simulink model "CANFDModel410_3"  (R2014a)
settings: Solver=ode45  StartTime=0.0  StopTime=200  RelTol=1e-3
undefined symbols (not defined in the file or in its folder): des, gcbh
undefined symbols (not defined in the file): BitR1, BitR2, DS, GEN_TIME
libraries: simeventslib x2, simulink x1
settings Model: Creator=PcMax  LastModifiedBy=PcMax

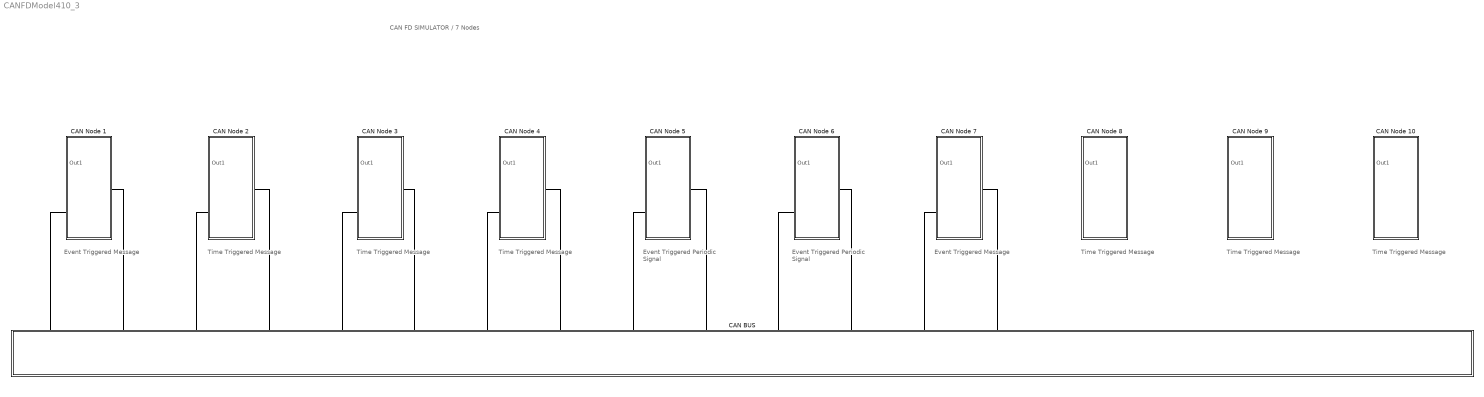
== system CANFDModel410_3 ==
  note: Event Triggered
      | Message
  note: CAN FD SIMULATOR / 7 Nodes
  note: Time Triggered
      | Message
  note: Event Triggered
      | Periodic Signal
  note: Time Triggered
      | Message
  note: Time Triggered
      | Message
  note: Event Triggered
      | Message
  note: Time Triggered
      | Message
  note: Time Triggered
      | Message
  note: Time Triggered
      | Message
  note: Event Triggered
      | Periodic Signal
  CAN BUS : Subsystem  mask{BitRate1=BitR1, BitRate2=BitR2, DSize=DS}
      mask prompts: BitRate1 "BitRate1 (Up to 1000 Kbit/s)"; BitRate2 "BitRate2 (Up to 8000 Kbit/s)"; DSize "DataSize (Up to 64 bytes)"
  CAN Node 1 : Subsystem  mask{Tint=GEN_TIME, Acc_ID=2, CAN_ID=1, bitlength=16, MAXM=800, MINM=400}
      mask prompts: Tint "Generation Time"; Acc_ID "Accepted CAN ID"; CAN_ID "Generation CAN ID"; bitlength "Bit Length"; MAXM "Message High"; MINM "Message Low"
  CAN Node 10 : Subsystem  mask{Tint=GEN_TIME, Acc_ID=2, CAN_ID=10, bitlength=16, MAXM=800, MINM=400}
      mask prompts: Tint "Generation Time"; Acc_ID "Accepted CAN ID"; CAN_ID "Generation CAN ID"; bitlength "Bit Length"; MAXM "Message High"; MINM "Message Low"
  CAN Node 2 : Subsystem  mask{Tint=GEN_TIME+5, Acc_ID=3, CAN_ID=2, bitlength=16, MAXM=800, MINM=400}
      mask prompts: Tint "Generation Time"; Acc_ID "Accepted CAN ID"; CAN_ID "Generation CAN ID"; bitlength "Bit Length"; MAXM "Message High"; MINM "Message Low"
  CAN Node 3 : Subsystem  mask{Tint=GEN_TIME+4, Acc_ID=2, CAN_ID=3, bitlength=16, MAXM=800, MINM=400}
      mask prompts: Tint "Generation Time"; Acc_ID "Accepted CAN ID"; CAN_ID "Generation CAN ID"; bitlength "Bit Length"; MAXM "Message High"; MINM "Message Low"
  CAN Node 4 : Subsystem  mask{Tint=GEN_TIME+3, Acc_ID=2, CAN_ID=4, bitlength=16, MAXM=800, MINM=400}
      mask prompts: Tint "Generation Time"; Acc_ID "Accepted CAN ID"; CAN_ID "Generation CAN ID"; bitlength "Bit Length"; MAXM "Message High"; MINM "Message Low"
  CAN Node 5 : Subsystem  mask{Tint=GEN_TIME, Acc_ID=1, CAN_ID=5, bitlength=16, MAXM=800, MINM=400}
      mask prompts: Tint "Generation Time"; Acc_ID "Accepted CAN ID"; CAN_ID "Generation CAN ID"; bitlength "Bit Length"; MAXM "Message High"; MINM "Message Low"
  CAN Node 6 : Subsystem  mask{Tint=GEN_TIME, Acc_ID=1, CAN_ID=6, bitlength=16, MAXM=800, MINM=400}
      mask prompts: Tint "Generation Time"; Acc_ID "Accepted CAN ID"; CAN_ID "Generation CAN ID"; bitlength "Bit Length"; MAXM "Message High"; MINM "Message Low"
  CAN Node 7 : Subsystem  mask{Tint=GEN_TIME, Acc_ID=2, CAN_ID=7, bitlength=16, MAXM=800, MINM=400}
      mask prompts: Tint "Generation Time"; Acc_ID "Accepted CAN ID"; CAN_ID "Generation CAN ID"; bitlength "Bit Length"; MAXM "Message High"; MINM "Message Low"
  CAN Node 8 : Subsystem  mask{Tint=GEN_TIME+2, Acc_ID=4, CAN_ID=8, bitlength=16, MAXM=800, MINM=400}
      mask prompts: Tint "Generation Time"; Acc_ID "Accepted CAN ID"; CAN_ID "Generation CAN ID"; bitlength "Bit Length"; MAXM "Message High"; MINM "Message Low"
  CAN Node 9 : Subsystem  mask{Tint=GEN_TIME+1, Acc_ID=6, CAN_ID=9, bitlength=16, MAXM=800, MINM=400}
      mask prompts: Tint "Generation Time"; Acc_ID "Accepted CAN ID"; CAN_ID "Generation CAN ID"; bitlength "Bit Length"; MAXM "Message High"; MINM "Message Low"
  connections:
  CAN Node 1/RConn1 -- CAN BUS/LConn1
  CAN Node 1/LConn1 -- CAN BUS/LConn2
  CAN Node 2/LConn1 -- CAN BUS/LConn4
  CAN BUS/LConn6 -- CAN Node 3/LConn1
  CAN Node 2/RConn1 -- CAN BUS/LConn3
  CAN Node 3/RConn1 -- CAN BUS/LConn5
  CAN Node 4/RConn1 -- CAN BUS/LConn7
  CAN Node 4/LConn1 -- CAN BUS/LConn8
  CAN Node 5/RConn1 -- CAN BUS/LConn9
  CAN Node 5/LConn1 -- CAN BUS/LConn10
  CAN Node 6/RConn1 -- CAN BUS/LConn11
  CAN Node 6/LConn1 -- CAN BUS/LConn12
  CAN Node 7/RConn1 -- CAN BUS/LConn13
  CAN Node 7/LConn1 -- CAN BUS/LConn14

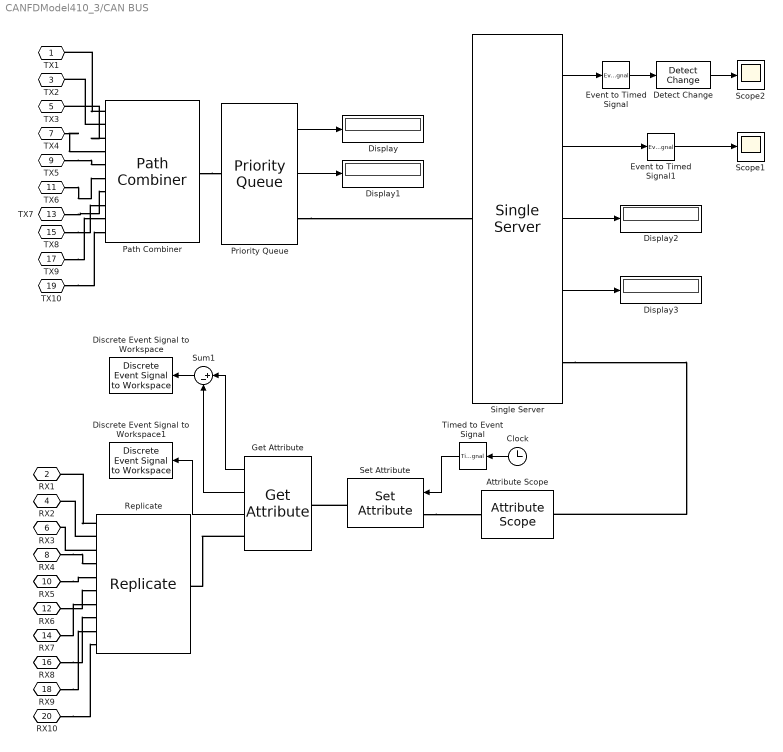
== system CANFDModel410_3/CAN BUS ==
  Attribute Scope : AttributeScope  LoadFcn=des.scope.CallbackSupport('seLoadFcn',gcbh)  StartFcn=des.scope.CallbackSupport('seStartFcn',gcbh)  StopFcn=des.scope.CallbackSupport('seStopFcn',gcbh)  PlotType=Stem  AttributeNameY=CAN_ID
      settings: CopyFcn=des.scope.CallbackSupport('seCopyFcn',gcbh)  DeleteFcn=des.scope.CallbackSupport('seDeleteFcn',gcbh)  PreSaveFcn=des.scope.CallbackSupport('sePreSaveFcn',gcbh)  NameChangeFcn=des.scope.CallbackSupport('seNameChangeFcn',gcbh)  OpenFcn=des.scope.CallbackSupport('seOpenFcn',gcbh)
  Clock : Clock
  Detect Change : simulink/Logic and Bit Operations/Detect Change  vinit=0  InputProcessing=Inherited  OutDataTypeStr=boolean
  Discrete Event Signal to Workspace : simeventslib/SimEvents Sinks/Discrete Event Signal to Workspace  VariableName=D  SaveFormat=Array  isMonitorOnly=off  isRecordIC=off
  Discrete Event Signal to Workspace1 : simeventslib/SimEvents Sinks/Discrete Event Signal to Workspace  VariableName=ID  SaveFormat=Array  isMonitorOnly=off  isRecordIC=off
  Display{,1..3} (4 alike) : Display
  Event to Timed Signal : EventToTimedSignal
  Event to Timed Signal1 : EventToTimedSignal
  Get Attribute : GetAttribute  AttributeName=Tim_arv|Tim_gen|CAN_ID  AttributeMissing=Error|Error|Error  AttributeDefaultValue=1|1|1  AttributeTreatAsVector=1|1|1  AttributeSendTiming=After entity departure|After entity departure|After entity departure  EvaluatedDefaultAttributeValue={ [];[];[]}
      settings: OutputPortMap=o1,o2,o3
  Path Combiner : PathCombiner  NumberInputPorts=10
  Priority Queue : PriorityQueue  Capacity=10  SortingAttributeName=CAN_ID  StatAverageWait=on  StatNumberTimedout=on
      settings: OutputPortMap=o2,o4
  Replicate : Replicate  NumberOutputPorts=10
  Scope1 : Scope
  Scope2 : Scope
      settings: SaveName=ScopeData2
  Set Attribute : SetAttribute  AttributeName=Tim_arv  AttributeFrom=Signal port  EvaluatedAttributeValue={ []}
  Single Server : SingleServer  ServiceTime=(32/BitRate1)+((28+10*DSize+17)/BitRate2)  StatNumberDeparted=on  StatNumberInBlock=on  StatAverageWait=on  StatUtilization=on
      settings: OutputPortMap=o0,o1,o4,o5
  Sum1 : Sum  Inputs=|+-
  Timed to Event Signal : TimedToEventSignal
  TX1 : PMIOPort  Port=1  Side=Left
  RX1 : PMIOPort  Port=2  Side=Left
  TX2 : PMIOPort  Port=3  Side=Left
  RX2 : PMIOPort  Port=4  Side=Left
  TX3 : PMIOPort  Port=5  Side=Left
  RX3 : PMIOPort  Port=6  Side=Left
  TX4 : PMIOPort  Port=7  Side=Left
  RX4 : PMIOPort  Port=8  Side=Left
  TX5 : PMIOPort  Port=9  Side=Left
  RX5 : PMIOPort  Port=10  Side=Left
  TX6 : PMIOPort  Port=11  Side=Left
  RX6 : PMIOPort  Port=12  Side=Left
  TX7 : PMIOPort  Port=13  Side=Left
  RX7 : PMIOPort  Port=14  Side=Left
  TX8 : PMIOPort  Port=15  Side=Left
  RX8 : PMIOPort  Port=16  Side=Left
  TX9 : PMIOPort  Port=17  Side=Left
  RX9 : PMIOPort  Port=18  Side=Left
  TX10 : PMIOPort  Port=19  Side=Left
  RX10 : PMIOPort  Port=20  Side=Left
  wires:
  Priority Queue/1 -> Display/1
  Single Server/4 -> Display3/1
  Single Server/1 -> Event to Timed Signal/1
  Single Server/2 -> Event to Timed Signal1/1
  Event to Timed Signal1/1 -> Scope1/1
  Priority Queue/2 -> Display1/1
  Single Server/3 -> Display2/1
  Event to Timed Signal/1 -> Detect Change/1
  Detect Change/1 -> Scope2/1
  Clock/1 -> Timed to Event Signal/1
  Timed to Event Signal/1 -> Set Attribute/1
  Get Attribute/1 -> Sum1/1
  Get Attribute/2 -> Sum1/2
  Get Attribute/3 -> Discrete Event Signal to Workspace1/1
  Sum1/1 -> Discrete Event Signal to Workspace/1
  connections:
  Path Combiner/LConn2 -- TX2/RConn1
  Replicate/RConn2 -- RX2/RConn1
  Path Combiner/LConn3 -- TX3/RConn1
  Replicate/RConn3 -- RX3/RConn1
  Path Combiner/LConn1 -- TX1/RConn1
  Replicate/RConn1 -- RX1/RConn1
  Priority Queue/RConn1 -- Single Server/LConn1
  Path Combiner/RConn1 -- Priority Queue/LConn1
  Single Server/RConn1 -- Attribute Scope/LConn1
  Set Attribute/LConn1 -- Attribute Scope/RConn1
  Set Attribute/RConn1 -- Get Attribute/LConn1
  Get Attribute/RConn1 -- Replicate/LConn1
  TX4/RConn1 -- Path Combiner/LConn4
  RX4/RConn1 -- Replicate/RConn4
  TX5/RConn1 -- Path Combiner/LConn5
  RX5/RConn1 -- Replicate/RConn5
  TX6/RConn1 -- Path Combiner/LConn6
  RX6/RConn1 -- Replicate/RConn6
  TX7/RConn1 -- Path Combiner/LConn7
  RX7/RConn1 -- Replicate/RConn7
  TX8/RConn1 -- Path Combiner/LConn8
  RX8/RConn1 -- Replicate/RConn8
  TX9/RConn1 -- Path Combiner/LConn9
  RX9/RConn1 -- Replicate/RConn9
  TX10/RConn1 -- Path Combiner/LConn10
  RX10/RConn1 -- Replicate/RConn10

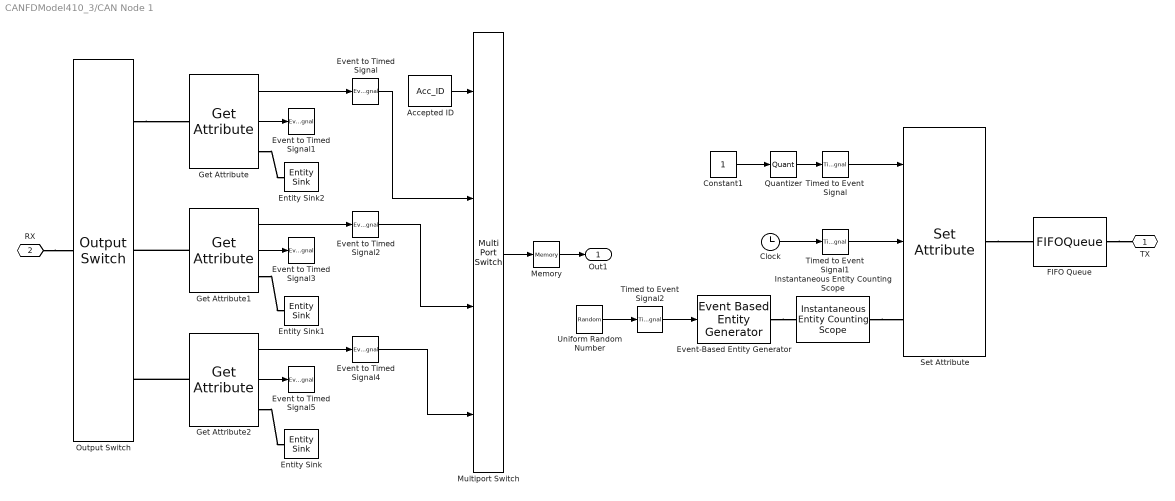
== system CANFDModel410_3/CAN Node 1 ==
  Accepted ID : Constant  Value=Acc_ID
  Clock : Clock
  Constant1 : Constant
  Entity Sink : EntitySink
  Entity Sink1 : EntitySink
  Entity Sink2 : EntitySink
  Event to Timed Signal{,1..5} (6 alike) : EventToTimedSignal
  Event-Based Entity Generator : EventBasedEntityGenerator
  FIFO Queue : FIFOQueue  Capacity=3
  Get Attribute : GetAttribute  AttributeName=Value|CAN_ID  AttributeMissing=Error|Error  AttributeDefaultValue=1|1  AttributeTreatAsVector=1|1  AttributeSendTiming=After entity departure|After entity departure  EvaluatedDefaultAttributeValue={ [];[]}
      settings: OutputPortMap=o1,o2
  Get Attribute1 : GetAttribute  AttributeName=Value|CAN_ID  AttributeMissing=Error|Error  AttributeDefaultValue=1|1  AttributeTreatAsVector=1|1  AttributeSendTiming=After entity departure|After entity departure  EvaluatedDefaultAttributeValue={ [];[]}
      settings: OutputPortMap=o1,o2
  Get Attribute2 : GetAttribute  AttributeName=Value|CAN_ID  AttributeMissing=Error|Error  AttributeDefaultValue=1|1  AttributeTreatAsVector=1|1  AttributeSendTiming=After entity departure|After entity departure  EvaluatedDefaultAttributeValue={ [];[]}
      settings: OutputPortMap=o1,o2
  Instantaneous Entity Counting Scope : InstantaneousEntityCountingScope  LoadFcn=des.scope.CallbackSupport('seLoadFcn',gcbh)  StartFcn=des.scope.CallbackSupport('seStartFcn',gcbh)  StopFcn=des.scope.CallbackSupport('seStopFcn',gcbh)
      settings: CopyFcn=des.scope.CallbackSupport('seCopyFcn',gcbh)  DeleteFcn=des.scope.CallbackSupport('seDeleteFcn',gcbh)  PreSaveFcn=des.scope.CallbackSupport('sePreSaveFcn',gcbh)  NameChangeFcn=des.scope.CallbackSupport('seNameChangeFcn',gcbh)  OpenFcn=des.scope.CallbackSupport('seOpenFcn',gcbh)
  Memory : Memory
  Multiport Switch : MultiPortSwitch
  Output Switch : OutputSwitch
  Quantizer : Quantizer  QuantizationInterval=(MAXM-MINM)/2^bitlength%%800/2^16%%
  Set Attribute : SetAttribute  AttributeName=Value|Tim_gen|CAN_ID  AttributeFrom=Signal port|Signal port|Dialog  AttributeValue=1|1|CAN_ID  AttributeTreatAsVector=1|1|1  EvaluatedAttributeValue={ [];[];CAN_ID}
      settings: InputPortMap=u0,u1
  Timed to Event Signal : TimedToEventSignal
  Timed to Event Signal1 : TimedToEventSignal
  Timed to Event Signal2 : TimedToEventSignal
  Uniform Random Number : UniformRandomNumber  SampleTime=Tint + 4
  TX : PMIOPort  Port=1  Side=Right
  RX : PMIOPort  Port=2  Side=Left
  Out1 : Outport
  wires:
  Quantizer/1 -> Timed to Event Signal/1
  Timed to Event Signal/1 -> Set Attribute/1
  Clock/1 -> Timed to Event Signal1/1
  Timed to Event Signal1/1 -> Set Attribute/2
  Constant1/1 -> Quantizer/1
  Get Attribute/2 -> Event to Timed Signal1/1
  Get Attribute/1 -> Event to Timed Signal/1
  Get Attribute1/1 -> Event to Timed Signal2/1
  Get Attribute1/2 -> Event to Timed Signal3/1
  Get Attribute2/1 -> Event to Timed Signal4/1
  Get Attribute2/2 -> Event to Timed Signal5/1
  Event to Timed Signal/1 -> Multiport Switch/2
  Event to Timed Signal2/1 -> Multiport Switch/3
  Event to Timed Signal4/1 -> Multiport Switch/4
  Accepted ID/1 -> Multiport Switch/1
  Multiport Switch/1 -> Memory/1
  Uniform Random Number/1 -> Timed to Event Signal2/1
  Timed to Event Signal2/1 -> Event-Based Entity Generator/1
  Memory/1 -> Out1/1
  connections:
  Set Attribute/RConn1 -- FIFO Queue/LConn1
  Event-Based Entity Generator/RConn1 -- Instantaneous Entity Counting Scope/LConn1
  FIFO Queue/RConn1 -- TX/RConn1
  RX/RConn1 -- Output Switch/LConn1
  Output Switch/RConn1 -- Get Attribute/LConn1
  Get Attribute1/LConn1 -- Output Switch/RConn2
  Get Attribute2/LConn1 -- Output Switch/RConn3
  Get Attribute2/RConn1 -- Entity Sink/LConn1
  Get Attribute/RConn1 -- Entity Sink2/LConn1
  Get Attribute1/RConn1 -- Entity Sink1/LConn1
  Instantaneous Entity Counting Scope/RConn1 -- Set Attribute/LConn1

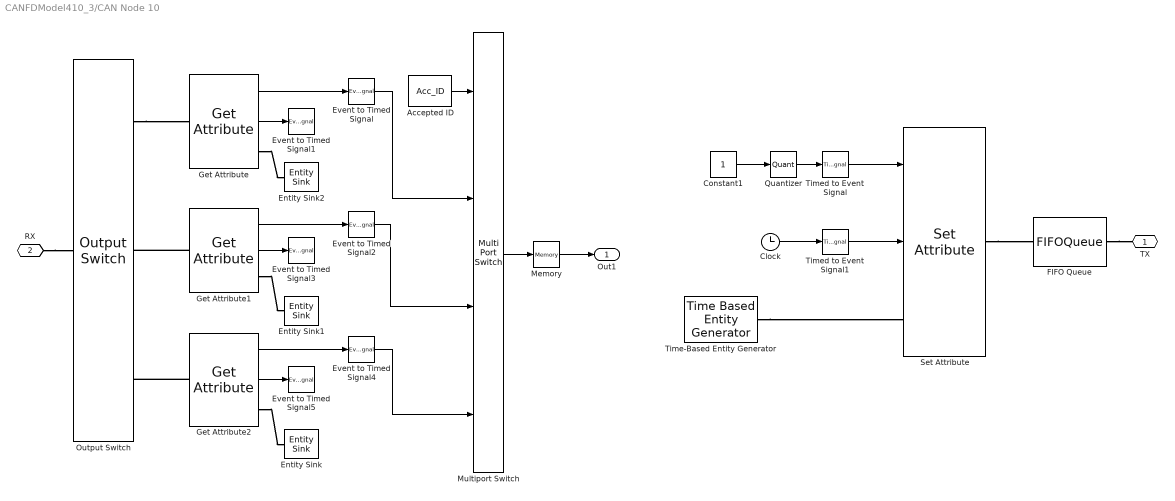
== system CANFDModel410_3/CAN Node 10 ==
  Accepted ID : Constant  Value=Acc_ID
  Clock : Clock
  Constant1 : Constant
  Entity Sink : EntitySink
  Entity Sink1 : EntitySink
  Entity Sink2 : EntitySink
  Event to Timed Signal{,1..5} (6 alike) : EventToTimedSignal
  FIFO Queue : FIFOQueue  Capacity=3
  Get Attribute : GetAttribute  AttributeName=Value|CAN_ID  AttributeMissing=Error|Error  AttributeDefaultValue=1|1  AttributeTreatAsVector=1|1  AttributeSendTiming=After entity departure|After entity departure  EvaluatedDefaultAttributeValue={ [];[]}
      settings: OutputPortMap=o1,o2
  Get Attribute1 : GetAttribute  AttributeName=Value|CAN_ID  AttributeMissing=Error|Error  AttributeDefaultValue=1|1  AttributeTreatAsVector=1|1  AttributeSendTiming=After entity departure|After entity departure  EvaluatedDefaultAttributeValue={ [];[]}
      settings: OutputPortMap=o1,o2
  Get Attribute2 : GetAttribute  AttributeName=Value|CAN_ID  AttributeMissing=Error|Error  AttributeDefaultValue=1|1  AttributeTreatAsVector=1|1  AttributeSendTiming=After entity departure|After entity departure  EvaluatedDefaultAttributeValue={ [];[]}
      settings: OutputPortMap=o1,o2
  Memory : Memory
  Multiport Switch : MultiPortSwitch
  Output Switch : OutputSwitch
  Quantizer : Quantizer  QuantizationInterval=(MAXM-MINM)/2^bitlength%%800/2^16%%
  Set Attribute : SetAttribute  AttributeName=Value|Tim_gen|CAN_ID  AttributeFrom=Signal port|Signal port|Dialog  AttributeValue=1|1|CAN_ID  AttributeTreatAsVector=1|1|1  EvaluatedAttributeValue={ [];[];CAN_ID}
      settings: InputPortMap=u0,u1
  Time-Based Entity Generator : TimeBasedEntityGenerator  Distribution=Uniform  Period=Tint  Minimum=Tint  Maximum=Tint+0.1
  Timed to Event Signal : TimedToEventSignal
  Timed to Event Signal1 : TimedToEventSignal
  TX : PMIOPort  Port=1  Side=Right
  RX : PMIOPort  Port=2  Side=Left
  Out1 : Outport
  wires:
  Quantizer/1 -> Timed to Event Signal/1
  Timed to Event Signal/1 -> Set Attribute/1
  Clock/1 -> Timed to Event Signal1/1
  Timed to Event Signal1/1 -> Set Attribute/2
  Constant1/1 -> Quantizer/1
  Get Attribute/2 -> Event to Timed Signal1/1
  Get Attribute/1 -> Event to Timed Signal/1
  Get Attribute1/1 -> Event to Timed Signal2/1
  Get Attribute1/2 -> Event to Timed Signal3/1
  Get Attribute2/1 -> Event to Timed Signal4/1
  Get Attribute2/2 -> Event to Timed Signal5/1
  Event to Timed Signal/1 -> Multiport Switch/2
  Event to Timed Signal2/1 -> Multiport Switch/3
  Event to Timed Signal4/1 -> Multiport Switch/4
  Accepted ID/1 -> Multiport Switch/1
  Multiport Switch/1 -> Memory/1
  Memory/1 -> Out1/1
  connections:
  Set Attribute/RConn1 -- FIFO Queue/LConn1
  Time-Based Entity Generator/RConn1 -- Set Attribute/LConn1
  FIFO Queue/RConn1 -- TX/RConn1
  RX/RConn1 -- Output Switch/LConn1
  Output Switch/RConn1 -- Get Attribute/LConn1
  Get Attribute1/LConn1 -- Output Switch/RConn2
  Get Attribute2/LConn1 -- Output Switch/RConn3
  Get Attribute2/RConn1 -- Entity Sink/LConn1
  Get Attribute/RConn1 -- Entity Sink2/LConn1
  Get Attribute1/RConn1 -- Entity Sink1/LConn1

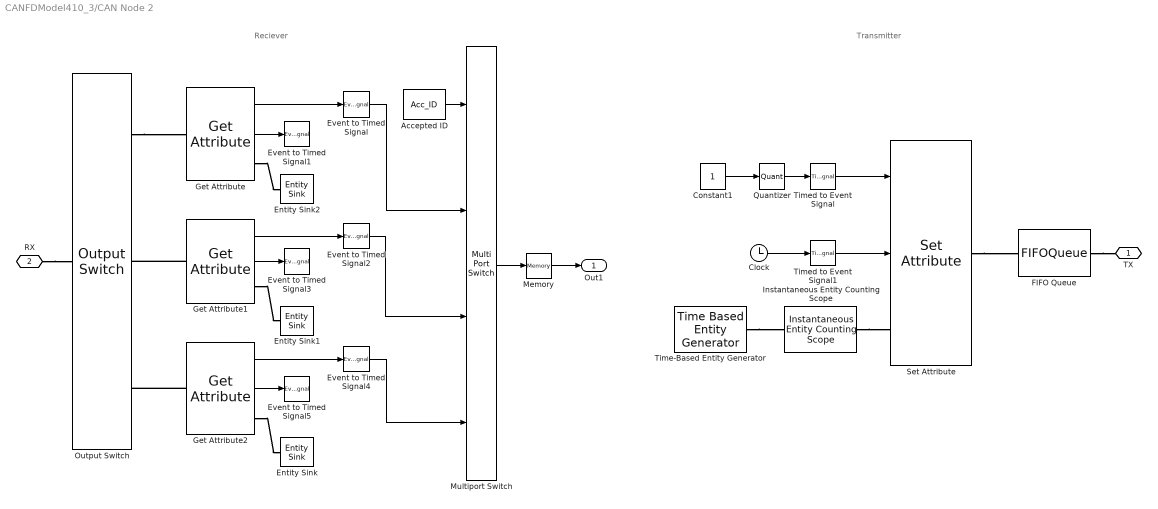
== system CANFDModel410_3/CAN Node 2 ==
  note: Reciever
  note: Transmitter
  Accepted ID : Constant  Value=Acc_ID
  Clock : Clock
  Constant1 : Constant
  Entity Sink : EntitySink
  Entity Sink1 : EntitySink
  Entity Sink2 : EntitySink
  Event to Timed Signal{,1..5} (6 alike) : EventToTimedSignal
  FIFO Queue : FIFOQueue  Capacity=3
  Get Attribute : GetAttribute  AttributeName=Value|CAN_ID  AttributeMissing=Error|Error  AttributeDefaultValue=1|1  AttributeTreatAsVector=1|1  AttributeSendTiming=After entity departure|After entity departure  EvaluatedDefaultAttributeValue={ [];[]}
      settings: OutputPortMap=o1,o2
  Get Attribute1 : GetAttribute  AttributeName=Value|CAN_ID  AttributeMissing=Error|Error  AttributeDefaultValue=1|1  AttributeTreatAsVector=1|1  AttributeSendTiming=After entity departure|After entity departure  EvaluatedDefaultAttributeValue={ [];[]}
      settings: OutputPortMap=o1,o2
  Get Attribute2 : GetAttribute  AttributeName=Value|CAN_ID  AttributeMissing=Error|Error  AttributeDefaultValue=1|1  AttributeTreatAsVector=1|1  AttributeSendTiming=After entity departure|After entity departure  EvaluatedDefaultAttributeValue={ [];[]}
      settings: OutputPortMap=o1,o2
  Instantaneous Entity Counting Scope : InstantaneousEntityCountingScope  LoadFcn=des.scope.CallbackSupport('seLoadFcn',gcbh)  StartFcn=des.scope.CallbackSupport('seStartFcn',gcbh)  StopFcn=des.scope.CallbackSupport('seStopFcn',gcbh)
      settings: CopyFcn=des.scope.CallbackSupport('seCopyFcn',gcbh)  DeleteFcn=des.scope.CallbackSupport('seDeleteFcn',gcbh)  PreSaveFcn=des.scope.CallbackSupport('sePreSaveFcn',gcbh)  NameChangeFcn=des.scope.CallbackSupport('seNameChangeFcn',gcbh)  OpenFcn=des.scope.CallbackSupport('seOpenFcn',gcbh)
  Memory : Memory
  Multiport Switch : MultiPortSwitch
  Output Switch : OutputSwitch
  Quantizer : Quantizer  QuantizationInterval=(MAXM-MINM)/2^bitlength%%800/2^16%%
  Set Attribute : SetAttribute  AttributeName=Value|Tim_gen|CAN_ID  AttributeFrom=Signal port|Signal port|Dialog  AttributeValue=1|1|CAN_ID  AttributeTreatAsVector=1|1|1  EvaluatedAttributeValue={ [];[];CAN_ID}
      settings: InputPortMap=u0,u1
  Time-Based Entity Generator : TimeBasedEntityGenerator  Distribution=Uniform  Period=Tint  Minimum=Tint  Maximum=Tint+0.1
  Timed to Event Signal : TimedToEventSignal
  Timed to Event Signal1 : TimedToEventSignal
  TX : PMIOPort  Port=1  Side=Right
  RX : PMIOPort  Port=2  Side=Left
  Out1 : Outport
  wires:
  Memory/1 -> Out1/1
  Multiport Switch/1 -> Memory/1
  Accepted ID/1 -> Multiport Switch/1
  Event to Timed Signal4/1 -> Multiport Switch/4
  Event to Timed Signal2/1 -> Multiport Switch/3
  Event to Timed Signal/1 -> Multiport Switch/2
  Get Attribute2/2 -> Event to Timed Signal5/1
  Get Attribute2/1 -> Event to Timed Signal4/1
  Get Attribute1/2 -> Event to Timed Signal3/1
  Get Attribute1/1 -> Event to Timed Signal2/1
  Get Attribute/1 -> Event to Timed Signal/1
  Get Attribute/2 -> Event to Timed Signal1/1
  Constant1/1 -> Quantizer/1
  Timed to Event Signal1/1 -> Set Attribute/2
  Clock/1 -> Timed to Event Signal1/1
  Timed to Event Signal/1 -> Set Attribute/1
  Quantizer/1 -> Timed to Event Signal/1
  connections:
  Get Attribute1/RConn1 -- Entity Sink1/LConn1
  Get Attribute/RConn1 -- Entity Sink2/LConn1
  Get Attribute2/RConn1 -- Entity Sink/LConn1
  Get Attribute2/LConn1 -- Output Switch/RConn3
  Get Attribute1/LConn1 -- Output Switch/RConn2
  Output Switch/RConn1 -- Get Attribute/LConn1
  RX/RConn1 -- Output Switch/LConn1
  FIFO Queue/RConn1 -- TX/RConn1
  Time-Based Entity Generator/RConn1 -- Instantaneous Entity Counting Scope/LConn1
  Set Attribute/RConn1 -- FIFO Queue/LConn1
  Instantaneous Entity Counting Scope/RConn1 -- Set Attribute/LConn1

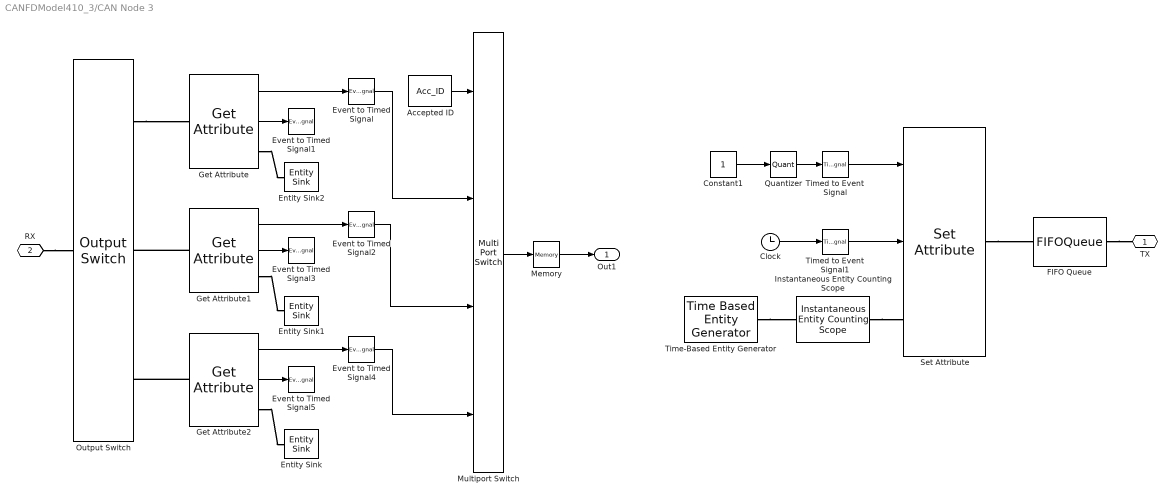
== system CANFDModel410_3/CAN Node 3 ==
  Accepted ID : Constant  Value=Acc_ID
  Clock : Clock
  Constant1 : Constant
  Entity Sink : EntitySink
  Entity Sink1 : EntitySink
  Entity Sink2 : EntitySink
  Event to Timed Signal{,1..5} (6 alike) : EventToTimedSignal
  FIFO Queue : FIFOQueue  Capacity=3
  Get Attribute : GetAttribute  AttributeName=Value|CAN_ID  AttributeMissing=Error|Error  AttributeDefaultValue=1|1  AttributeTreatAsVector=1|1  AttributeSendTiming=After entity departure|After entity departure  EvaluatedDefaultAttributeValue={ [];[]}
      settings: OutputPortMap=o1,o2
  Get Attribute1 : GetAttribute  AttributeName=Value|CAN_ID  AttributeMissing=Error|Error  AttributeDefaultValue=1|1  AttributeTreatAsVector=1|1  AttributeSendTiming=After entity departure|After entity departure  EvaluatedDefaultAttributeValue={ [];[]}
      settings: OutputPortMap=o1,o2
  Get Attribute2 : GetAttribute  AttributeName=Value|CAN_ID  AttributeMissing=Error|Error  AttributeDefaultValue=1|1  AttributeTreatAsVector=1|1  AttributeSendTiming=After entity departure|After entity departure  EvaluatedDefaultAttributeValue={ [];[]}
      settings: OutputPortMap=o1,o2
  Instantaneous Entity Counting Scope : InstantaneousEntityCountingScope  LoadFcn=des.scope.CallbackSupport('seLoadFcn',gcbh)  StartFcn=des.scope.CallbackSupport('seStartFcn',gcbh)  StopFcn=des.scope.CallbackSupport('seStopFcn',gcbh)
      settings: CopyFcn=des.scope.CallbackSupport('seCopyFcn',gcbh)  DeleteFcn=des.scope.CallbackSupport('seDeleteFcn',gcbh)  PreSaveFcn=des.scope.CallbackSupport('sePreSaveFcn',gcbh)  NameChangeFcn=des.scope.CallbackSupport('seNameChangeFcn',gcbh)  OpenFcn=des.scope.CallbackSupport('seOpenFcn',gcbh)
  Memory : Memory
  Multiport Switch : MultiPortSwitch
  Output Switch : OutputSwitch
  Quantizer : Quantizer  QuantizationInterval=(MAXM-MINM)/2^bitlength%%800/2^16%%
  Set Attribute : SetAttribute  AttributeName=Value|Tim_gen|CAN_ID  AttributeFrom=Signal port|Signal port|Dialog  AttributeValue=1|1|CAN_ID  AttributeTreatAsVector=1|1|1  EvaluatedAttributeValue={ [];[];CAN_ID}
      settings: InputPortMap=u0,u1
  Time-Based Entity Generator : TimeBasedEntityGenerator  Distribution=Uniform  Period=Tint  Minimum=Tint  Maximum=Tint+0.1
  Timed to Event Signal : TimedToEventSignal
  Timed to Event Signal1 : TimedToEventSignal
  TX : PMIOPort  Port=1  Side=Right
  RX : PMIOPort  Port=2  Side=Left
  Out1 : Outport
  wires:
  Quantizer/1 -> Timed to Event Signal/1
  Timed to Event Signal/1 -> Set Attribute/1
  Clock/1 -> Timed to Event Signal1/1
  Timed to Event Signal1/1 -> Set Attribute/2
  Constant1/1 -> Quantizer/1
  Get Attribute/2 -> Event to Timed Signal1/1
  Get Attribute/1 -> Event to Timed Signal/1
  Get Attribute1/1 -> Event to Timed Signal2/1
  Get Attribute1/2 -> Event to Timed Signal3/1
  Get Attribute2/1 -> Event to Timed Signal4/1
  Get Attribute2/2 -> Event to Timed Signal5/1
  Event to Timed Signal/1 -> Multiport Switch/2
  Event to Timed Signal2/1 -> Multiport Switch/3
  Event to Timed Signal4/1 -> Multiport Switch/4
  Accepted ID/1 -> Multiport Switch/1
  Multiport Switch/1 -> Memory/1
  Memory/1 -> Out1/1
  connections:
  Set Attribute/RConn1 -- FIFO Queue/LConn1
  Time-Based Entity Generator/RConn1 -- Instantaneous Entity Counting Scope/LConn1
  FIFO Queue/RConn1 -- TX/RConn1
  RX/RConn1 -- Output Switch/LConn1
  Output Switch/RConn1 -- Get Attribute/LConn1
  Get Attribute1/LConn1 -- Output Switch/RConn2
  Get Attribute2/LConn1 -- Output Switch/RConn3
  Get Attribute2/RConn1 -- Entity Sink/LConn1
  Get Attribute/RConn1 -- Entity Sink2/LConn1
  Get Attribute1/RConn1 -- Entity Sink1/LConn1
  Instantaneous Entity Counting Scope/RConn1 -- Set Attribute/LConn1

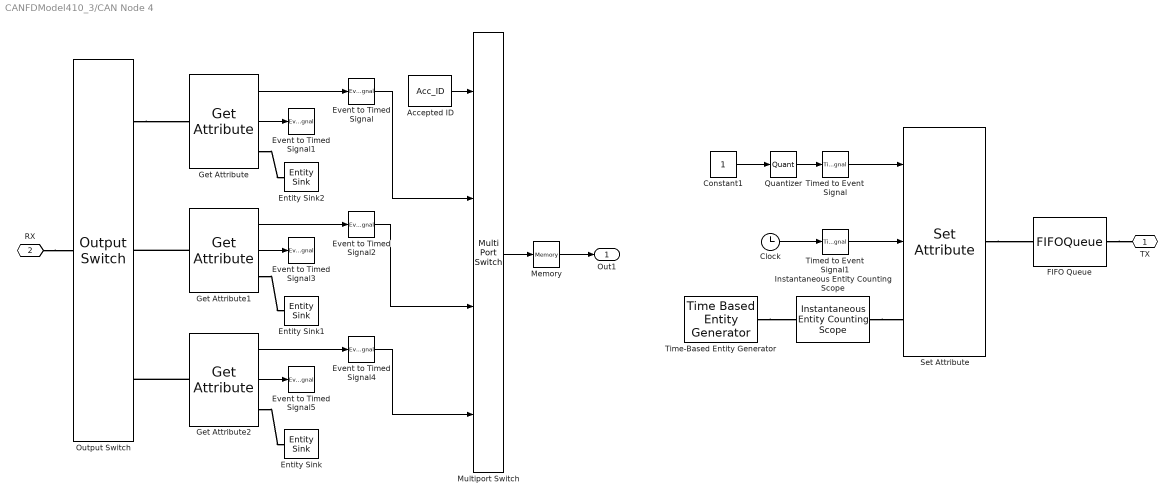
== system CANFDModel410_3/CAN Node 4 ==
  Accepted ID : Constant  Value=Acc_ID
  Clock : Clock
  Constant1 : Constant
  Entity Sink : EntitySink
  Entity Sink1 : EntitySink
  Entity Sink2 : EntitySink
  Event to Timed Signal{,1..5} (6 alike) : EventToTimedSignal
  FIFO Queue : FIFOQueue  Capacity=3
  Get Attribute : GetAttribute  AttributeName=Value|CAN_ID  AttributeMissing=Error|Error  AttributeDefaultValue=1|1  AttributeTreatAsVector=1|1  AttributeSendTiming=After entity departure|After entity departure  EvaluatedDefaultAttributeValue={ [];[]}
      settings: OutputPortMap=o1,o2
  Get Attribute1 : GetAttribute  AttributeName=Value|CAN_ID  AttributeMissing=Error|Error  AttributeDefaultValue=1|1  AttributeTreatAsVector=1|1  AttributeSendTiming=After entity departure|After entity departure  EvaluatedDefaultAttributeValue={ [];[]}
      settings: OutputPortMap=o1,o2
  Get Attribute2 : GetAttribute  AttributeName=Value|CAN_ID  AttributeMissing=Error|Error  AttributeDefaultValue=1|1  AttributeTreatAsVector=1|1  AttributeSendTiming=After entity departure|After entity departure  EvaluatedDefaultAttributeValue={ [];[]}
      settings: OutputPortMap=o1,o2
  Instantaneous Entity Counting Scope : InstantaneousEntityCountingScope  LoadFcn=des.scope.CallbackSupport('seLoadFcn',gcbh)  StartFcn=des.scope.CallbackSupport('seStartFcn',gcbh)  StopFcn=des.scope.CallbackSupport('seStopFcn',gcbh)
      settings: CopyFcn=des.scope.CallbackSupport('seCopyFcn',gcbh)  DeleteFcn=des.scope.CallbackSupport('seDeleteFcn',gcbh)  PreSaveFcn=des.scope.CallbackSupport('sePreSaveFcn',gcbh)  NameChangeFcn=des.scope.CallbackSupport('seNameChangeFcn',gcbh)  OpenFcn=des.scope.CallbackSupport('seOpenFcn',gcbh)
  Memory : Memory
  Multiport Switch : MultiPortSwitch
  Output Switch : OutputSwitch
  Quantizer : Quantizer  QuantizationInterval=(MAXM-MINM)/2^bitlength%%800/2^16%%
  Set Attribute : SetAttribute  AttributeName=Value|Tim_gen|CAN_ID  AttributeFrom=Signal port|Signal port|Dialog  AttributeValue=1|1|CAN_ID  AttributeTreatAsVector=1|1|1  EvaluatedAttributeValue={ [];[];CAN_ID}
      settings: InputPortMap=u0,u1
  Time-Based Entity Generator : TimeBasedEntityGenerator  Distribution=Uniform  Period=Tint  Minimum=Tint  Maximum=Tint+0.1
  Timed to Event Signal : TimedToEventSignal
  Timed to Event Signal1 : TimedToEventSignal
  TX : PMIOPort  Port=1  Side=Right
  RX : PMIOPort  Port=2  Side=Left
  Out1 : Outport
  wires:
  Memory/1 -> Out1/1
  Multiport Switch/1 -> Memory/1
  Accepted ID/1 -> Multiport Switch/1
  Event to Timed Signal4/1 -> Multiport Switch/4
  Event to Timed Signal2/1 -> Multiport Switch/3
  Event to Timed Signal/1 -> Multiport Switch/2
  Get Attribute2/2 -> Event to Timed Signal5/1
  Get Attribute2/1 -> Event to Timed Signal4/1
  Get Attribute1/2 -> Event to Timed Signal3/1
  Get Attribute1/1 -> Event to Timed Signal2/1
  Get Attribute/1 -> Event to Timed Signal/1
  Get Attribute/2 -> Event to Timed Signal1/1
  Constant1/1 -> Quantizer/1
  Timed to Event Signal1/1 -> Set Attribute/2
  Clock/1 -> Timed to Event Signal1/1
  Timed to Event Signal/1 -> Set Attribute/1
  Quantizer/1 -> Timed to Event Signal/1
  connections:
  Get Attribute1/RConn1 -- Entity Sink1/LConn1
  Get Attribute/RConn1 -- Entity Sink2/LConn1
  Get Attribute2/RConn1 -- Entity Sink/LConn1
  Get Attribute2/LConn1 -- Output Switch/RConn3
  Get Attribute1/LConn1 -- Output Switch/RConn2
  Output Switch/RConn1 -- Get Attribute/LConn1
  RX/RConn1 -- Output Switch/LConn1
  FIFO Queue/RConn1 -- TX/RConn1
  Instantaneous Entity Counting Scope/RConn1 -- Set Attribute/LConn1
  Set Attribute/RConn1 -- FIFO Queue/LConn1
  Time-Based Entity Generator/RConn1 -- Instantaneous Entity Counting Scope/LConn1

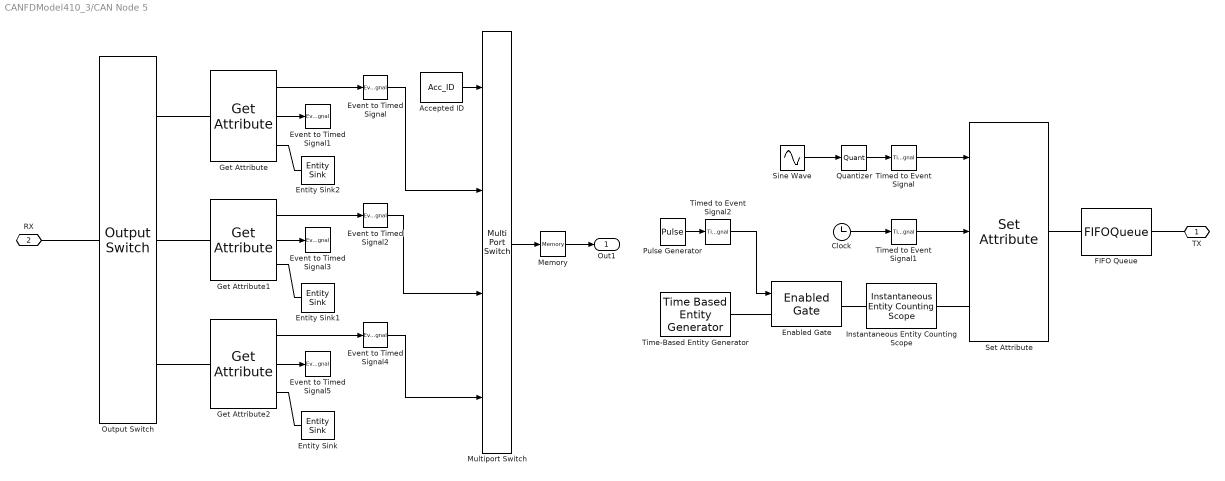
== system CANFDModel410_3/CAN Node 5 ==
  Accepted ID : Constant  Value=Acc_ID
  Clock : Clock
  Enabled Gate : EnabledGate
  Entity Sink : EntitySink
  Entity Sink1 : EntitySink
  Entity Sink2 : EntitySink
  Event to Timed Signal{,1..5} (6 alike) : EventToTimedSignal
  FIFO Queue : FIFOQueue  Capacity=3
  Get Attribute : GetAttribute  AttributeName=Value|Tim_gen  AttributeMissing=Error|Error  AttributeDefaultValue=1|1  AttributeTreatAsVector=1|1  AttributeSendTiming=After entity departure|After entity departure  EvaluatedDefaultAttributeValue={ [];[]}
      settings: OutputPortMap=o1,o2
  Get Attribute1 : GetAttribute  AttributeName=Value|Tim_gen  AttributeMissing=Error|Error  AttributeDefaultValue=1|1  AttributeTreatAsVector=1|1  AttributeSendTiming=After entity departure|After entity departure  EvaluatedDefaultAttributeValue={ [];[]}
      settings: OutputPortMap=o1,o2
  Get Attribute2 : GetAttribute  AttributeName=Value|Tim_gen  AttributeMissing=Error|Error  AttributeDefaultValue=1|1  AttributeTreatAsVector=1|1  AttributeSendTiming=After entity departure|After entity departure  EvaluatedDefaultAttributeValue={ [];[]}
      settings: OutputPortMap=o1,o2
  Instantaneous Entity Counting Scope : InstantaneousEntityCountingScope  LoadFcn=des.scope.CallbackSupport('seLoadFcn',gcbh)  StartFcn=des.scope.CallbackSupport('seStartFcn',gcbh)  StopFcn=des.scope.CallbackSupport('seStopFcn',gcbh)
      settings: CopyFcn=des.scope.CallbackSupport('seCopyFcn',gcbh)  DeleteFcn=des.scope.CallbackSupport('seDeleteFcn',gcbh)  PreSaveFcn=des.scope.CallbackSupport('sePreSaveFcn',gcbh)  NameChangeFcn=des.scope.CallbackSupport('seNameChangeFcn',gcbh)  OpenFcn=des.scope.CallbackSupport('seOpenFcn',gcbh)
  Memory : Memory
  Multiport Switch : MultiPortSwitch
  Output Switch : OutputSwitch
  Pulse Generator : DiscretePulseGenerator  Period=50  PulseWidth=30  PhaseDelay=3  VectorParams1D=off
  Quantizer : Quantizer  QuantizationInterval=(MAXM-MINM)/2^bitlength%%800/2^16%%
  Set Attribute : SetAttribute  AttributeName=Value|Tim_gen|CAN_ID  AttributeFrom=Signal port|Signal port|Dialog  AttributeValue=1|1|CAN_ID  AttributeTreatAsVector=1|1|1  EvaluatedAttributeValue={ [];[];CAN_ID}
      settings: InputPortMap=u0,u1
  Sine Wave : Sin  SampleTime=0
  Time-Based Entity Generator : TimeBasedEntityGenerator  Distribution=Uniform  Period=Tint  Minimum=Tint  Maximum=Tint+0.1  ResponseWhenUnblocked=Delayed restart
  Timed to Event Signal : TimedToEventSignal
  Timed to Event Signal1 : TimedToEventSignal
  Timed to Event Signal2 : TimedToEventSignal
  TX : PMIOPort  Port=1  Side=Right
  RX : PMIOPort  Port=2  Side=Left
  Out1 : Outport
  wires:
  Pulse Generator/1 -> Timed to Event Signal2/1
  Timed to Event Signal2/1 -> Enabled Gate/1
  Quantizer/1 -> Timed to Event Signal/1
  Timed to Event Signal/1 -> Set Attribute/1
  Clock/1 -> Timed to Event Signal1/1
  Timed to Event Signal1/1 -> Set Attribute/2
  Sine Wave/1 -> Quantizer/1
  Get Attribute/2 -> Event to Timed Signal1/1
  Get Attribute/1 -> Event to Timed Signal/1
  Get Attribute1/1 -> Event to Timed Signal2/1
  Get Attribute1/2 -> Event to Timed Signal3/1
  Get Attribute2/1 -> Event to Timed Signal4/1
  Get Attribute2/2 -> Event to Timed Signal5/1
  Event to Timed Signal/1 -> Multiport Switch/2
  Event to Timed Signal2/1 -> Multiport Switch/3
  Event to Timed Signal4/1 -> Multiport Switch/4
  Accepted ID/1 -> Multiport Switch/1
  Multiport Switch/1 -> Memory/1
  Memory/1 -> Out1/1
  connections:
  Time-Based Entity Generator/RConn1 -- Enabled Gate/LConn1
  RX/RConn1 -- Output Switch/LConn1
  Set Attribute/RConn1 -- FIFO Queue/LConn1
  Instantaneous Entity Counting Scope/LConn1 -- Enabled Gate/RConn1
  FIFO Queue/RConn1 -- TX/RConn1
  Output Switch/RConn1 -- Get Attribute/LConn1
  Get Attribute1/LConn1 -- Output Switch/RConn2
  Get Attribute2/LConn1 -- Output Switch/RConn3
  Get Attribute2/RConn1 -- Entity Sink/LConn1
  Get Attribute/RConn1 -- Entity Sink2/LConn1
  Get Attribute1/RConn1 -- Entity Sink1/LConn1
  Instantaneous Entity Counting Scope/RConn1 -- Set Attribute/LConn1

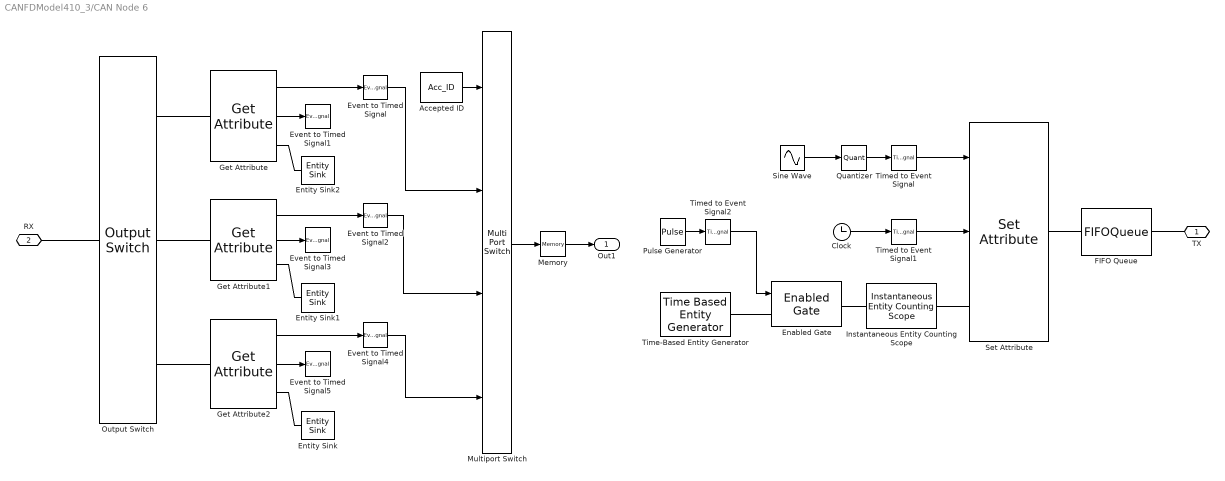
== system CANFDModel410_3/CAN Node 6 ==
  Accepted ID : Constant  Value=Acc_ID
  Clock : Clock
  Enabled Gate : EnabledGate
  Entity Sink : EntitySink
  Entity Sink1 : EntitySink
  Entity Sink2 : EntitySink
  Event to Timed Signal{,1..5} (6 alike) : EventToTimedSignal
  FIFO Queue : FIFOQueue  Capacity=3
  Get Attribute : GetAttribute  AttributeName=Value|Tim_gen  AttributeMissing=Error|Error  AttributeDefaultValue=1|1  AttributeTreatAsVector=1|1  AttributeSendTiming=After entity departure|After entity departure  EvaluatedDefaultAttributeValue={ [];[]}
      settings: OutputPortMap=o1,o2
  Get Attribute1 : GetAttribute  AttributeName=Value|Tim_gen  AttributeMissing=Error|Error  AttributeDefaultValue=1|1  AttributeTreatAsVector=1|1  AttributeSendTiming=After entity departure|After entity departure  EvaluatedDefaultAttributeValue={ [];[]}
      settings: OutputPortMap=o1,o2
  Get Attribute2 : GetAttribute  AttributeName=Value|Tim_gen  AttributeMissing=Error|Error  AttributeDefaultValue=1|1  AttributeTreatAsVector=1|1  AttributeSendTiming=After entity departure|After entity departure  EvaluatedDefaultAttributeValue={ [];[]}
      settings: OutputPortMap=o1,o2
  Instantaneous Entity Counting Scope : InstantaneousEntityCountingScope  LoadFcn=des.scope.CallbackSupport('seLoadFcn',gcbh)  StartFcn=des.scope.CallbackSupport('seStartFcn',gcbh)  StopFcn=des.scope.CallbackSupport('seStopFcn',gcbh)
      settings: CopyFcn=des.scope.CallbackSupport('seCopyFcn',gcbh)  DeleteFcn=des.scope.CallbackSupport('seDeleteFcn',gcbh)  PreSaveFcn=des.scope.CallbackSupport('sePreSaveFcn',gcbh)  NameChangeFcn=des.scope.CallbackSupport('seNameChangeFcn',gcbh)  OpenFcn=des.scope.CallbackSupport('seOpenFcn',gcbh)
  Memory : Memory
  Multiport Switch : MultiPortSwitch
  Output Switch : OutputSwitch
  Pulse Generator : DiscretePulseGenerator  Period=50  PulseWidth=30  PhaseDelay=3  VectorParams1D=off
  Quantizer : Quantizer  QuantizationInterval=(MAXM-MINM)/2^bitlength%%800/2^16%%
  Set Attribute : SetAttribute  AttributeName=Value|Tim_gen|CAN_ID  AttributeFrom=Signal port|Signal port|Dialog  AttributeValue=1|1|CAN_ID  AttributeTreatAsVector=1|1|1  EvaluatedAttributeValue={ [];[];CAN_ID}
      settings: InputPortMap=u0,u1
  Sine Wave : Sin  SampleTime=0
  Time-Based Entity Generator : TimeBasedEntityGenerator  Distribution=Uniform  Period=Tint  Minimum=Tint  Maximum=Tint+0.1  ResponseWhenUnblocked=Delayed restart
  Timed to Event Signal : TimedToEventSignal
  Timed to Event Signal1 : TimedToEventSignal
  Timed to Event Signal2 : TimedToEventSignal
  TX : PMIOPort  Port=1  Side=Right
  RX : PMIOPort  Port=2  Side=Left
  Out1 : Outport
  wires:
  Memory/1 -> Out1/1
  Multiport Switch/1 -> Memory/1
  Accepted ID/1 -> Multiport Switch/1
  Event to Timed Signal4/1 -> Multiport Switch/4
  Event to Timed Signal2/1 -> Multiport Switch/3
  Event to Timed Signal/1 -> Multiport Switch/2
  Get Attribute2/2 -> Event to Timed Signal5/1
  Get Attribute2/1 -> Event to Timed Signal4/1
  Get Attribute1/2 -> Event to Timed Signal3/1
  Get Attribute1/1 -> Event to Timed Signal2/1
  Get Attribute/1 -> Event to Timed Signal/1
  Get Attribute/2 -> Event to Timed Signal1/1
  Sine Wave/1 -> Quantizer/1
  Timed to Event Signal1/1 -> Set Attribute/2
  Clock/1 -> Timed to Event Signal1/1
  Timed to Event Signal/1 -> Set Attribute/1
  Quantizer/1 -> Timed to Event Signal/1
  Timed to Event Signal2/1 -> Enabled Gate/1
  Pulse Generator/1 -> Timed to Event Signal2/1
  connections:
  Instantaneous Entity Counting Scope/RConn1 -- Set Attribute/LConn1
  Get Attribute1/RConn1 -- Entity Sink1/LConn1
  Get Attribute/RConn1 -- Entity Sink2/LConn1
  Get Attribute2/RConn1 -- Entity Sink/LConn1
  Get Attribute2/LConn1 -- Output Switch/RConn3
  Get Attribute1/LConn1 -- Output Switch/RConn2
  Output Switch/RConn1 -- Get Attribute/LConn1
  FIFO Queue/RConn1 -- TX/RConn1
  Instantaneous Entity Counting Scope/LConn1 -- Enabled Gate/RConn1
  Set Attribute/RConn1 -- FIFO Queue/LConn1
  RX/RConn1 -- Output Switch/LConn1
  Time-Based Entity Generator/RConn1 -- Enabled Gate/LConn1

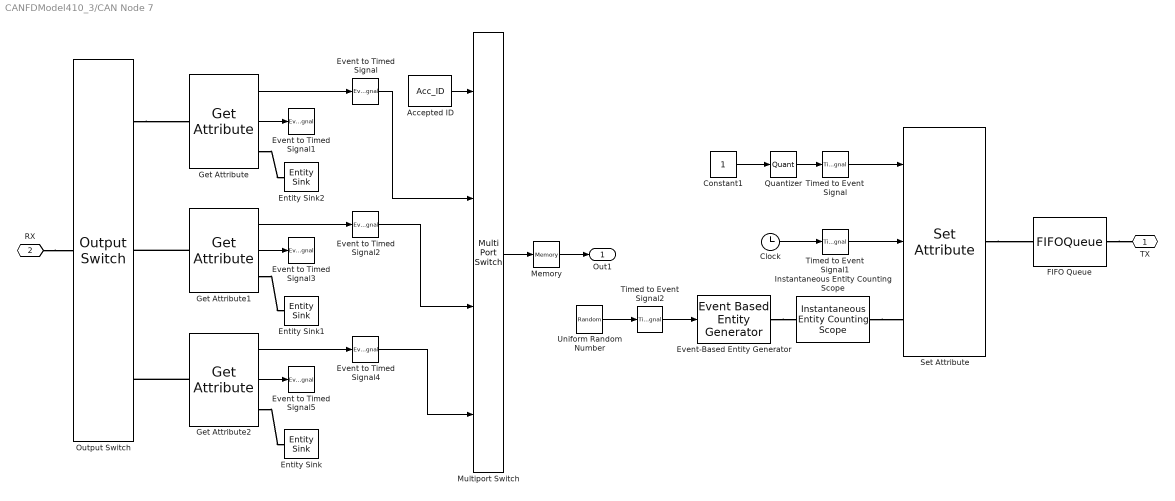
== system CANFDModel410_3/CAN Node 7 ==
  Accepted ID : Constant  Value=Acc_ID
  Clock : Clock
  Constant1 : Constant
  Entity Sink : EntitySink
  Entity Sink1 : EntitySink
  Entity Sink2 : EntitySink
  Event to Timed Signal{,1..5} (6 alike) : EventToTimedSignal
  Event-Based Entity Generator : EventBasedEntityGenerator
  FIFO Queue : FIFOQueue  Capacity=3
  Get Attribute : GetAttribute  AttributeName=Value|CAN_ID  AttributeMissing=Error|Error  AttributeDefaultValue=1|1  AttributeTreatAsVector=1|1  AttributeSendTiming=After entity departure|After entity departure  EvaluatedDefaultAttributeValue={ [];[]}
      settings: OutputPortMap=o1,o2
  Get Attribute1 : GetAttribute  AttributeName=Value|CAN_ID  AttributeMissing=Error|Error  AttributeDefaultValue=1|1  AttributeTreatAsVector=1|1  AttributeSendTiming=After entity departure|After entity departure  EvaluatedDefaultAttributeValue={ [];[]}
      settings: OutputPortMap=o1,o2
  Get Attribute2 : GetAttribute  AttributeName=Value|CAN_ID  AttributeMissing=Error|Error  AttributeDefaultValue=1|1  AttributeTreatAsVector=1|1  AttributeSendTiming=After entity departure|After entity departure  EvaluatedDefaultAttributeValue={ [];[]}
      settings: OutputPortMap=o1,o2
  Instantaneous Entity Counting Scope : InstantaneousEntityCountingScope  LoadFcn=des.scope.CallbackSupport('seLoadFcn',gcbh)  StartFcn=des.scope.CallbackSupport('seStartFcn',gcbh)  StopFcn=des.scope.CallbackSupport('seStopFcn',gcbh)
      settings: CopyFcn=des.scope.CallbackSupport('seCopyFcn',gcbh)  DeleteFcn=des.scope.CallbackSupport('seDeleteFcn',gcbh)  PreSaveFcn=des.scope.CallbackSupport('sePreSaveFcn',gcbh)  NameChangeFcn=des.scope.CallbackSupport('seNameChangeFcn',gcbh)  OpenFcn=des.scope.CallbackSupport('seOpenFcn',gcbh)
  Memory : Memory
  Multiport Switch : MultiPortSwitch
  Output Switch : OutputSwitch
  Quantizer : Quantizer  QuantizationInterval=(MAXM-MINM)/2^bitlength%%800/2^16%%
  Set Attribute : SetAttribute  AttributeName=Value|Tim_gen|CAN_ID  AttributeFrom=Signal port|Signal port|Dialog  AttributeValue=1|1|CAN_ID  AttributeTreatAsVector=1|1|1  EvaluatedAttributeValue={ [];[];CAN_ID}
      settings: InputPortMap=u0,u1
  Timed to Event Signal : TimedToEventSignal
  Timed to Event Signal1 : TimedToEventSignal
  Timed to Event Signal2 : TimedToEventSignal
  Uniform Random Number : UniformRandomNumber  SampleTime=Tint + 2
  TX : PMIOPort  Port=1  Side=Right
  RX : PMIOPort  Port=2  Side=Left
  Out1 : Outport
  wires:
  Timed to Event Signal2/1 -> Event-Based Entity Generator/1
  Uniform Random Number/1 -> Timed to Event Signal2/1
  Memory/1 -> Out1/1
  Multiport Switch/1 -> Memory/1
  Accepted ID/1 -> Multiport Switch/1
  Event to Timed Signal4/1 -> Multiport Switch/4
  Event to Timed Signal2/1 -> Multiport Switch/3
  Event to Timed Signal/1 -> Multiport Switch/2
  Get Attribute2/2 -> Event to Timed Signal5/1
  Get Attribute2/1 -> Event to Timed Signal4/1
  Get Attribute1/2 -> Event to Timed Signal3/1
  Get Attribute1/1 -> Event to Timed Signal2/1
  Get Attribute/1 -> Event to Timed Signal/1
  Get Attribute/2 -> Event to Timed Signal1/1
  Constant1/1 -> Quantizer/1
  Timed to Event Signal1/1 -> Set Attribute/2
  Clock/1 -> Timed to Event Signal1/1
  Timed to Event Signal/1 -> Set Attribute/1
  Quantizer/1 -> Timed to Event Signal/1
  connections:
  Get Attribute1/RConn1 -- Entity Sink1/LConn1
  Get Attribute/RConn1 -- Entity Sink2/LConn1
  Get Attribute2/RConn1 -- Entity Sink/LConn1
  Get Attribute2/LConn1 -- Output Switch/RConn3
  Get Attribute1/LConn1 -- Output Switch/RConn2
  Output Switch/RConn1 -- Get Attribute/LConn1
  RX/RConn1 -- Output Switch/LConn1
  FIFO Queue/RConn1 -- TX/RConn1
  Event-Based Entity Generator/RConn1 -- Instantaneous Entity Counting Scope/LConn1
  Set Attribute/RConn1 -- FIFO Queue/LConn1
  Instantaneous Entity Counting Scope/RConn1 -- Set Attribute/LConn1

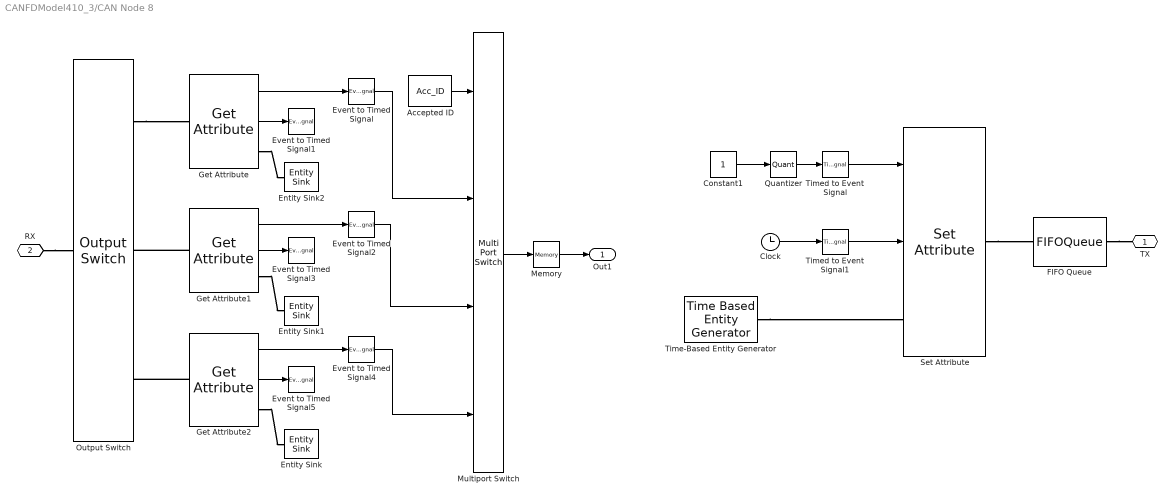
== system CANFDModel410_3/CAN Node 8 ==
  Accepted ID : Constant  Value=Acc_ID
  Clock : Clock
  Constant1 : Constant
  Entity Sink : EntitySink
  Entity Sink1 : EntitySink
  Entity Sink2 : EntitySink
  Event to Timed Signal{,1..5} (6 alike) : EventToTimedSignal
  FIFO Queue : FIFOQueue  Capacity=3
  Get Attribute : GetAttribute  AttributeName=Value|CAN_ID  AttributeMissing=Error|Error  AttributeDefaultValue=1|1  AttributeTreatAsVector=1|1  AttributeSendTiming=After entity departure|After entity departure  EvaluatedDefaultAttributeValue={ [];[]}
      settings: OutputPortMap=o1,o2
  Get Attribute1 : GetAttribute  AttributeName=Value|CAN_ID  AttributeMissing=Error|Error  AttributeDefaultValue=1|1  AttributeTreatAsVector=1|1  AttributeSendTiming=After entity departure|After entity departure  EvaluatedDefaultAttributeValue={ [];[]}
      settings: OutputPortMap=o1,o2
  Get Attribute2 : GetAttribute  AttributeName=Value|CAN_ID  AttributeMissing=Error|Error  AttributeDefaultValue=1|1  AttributeTreatAsVector=1|1  AttributeSendTiming=After entity departure|After entity departure  EvaluatedDefaultAttributeValue={ [];[]}
      settings: OutputPortMap=o1,o2
  Memory : Memory
  Multiport Switch : MultiPortSwitch
  Output Switch : OutputSwitch
  Quantizer : Quantizer  QuantizationInterval=(MAXM-MINM)/2^bitlength%%800/2^16%%
  Set Attribute : SetAttribute  AttributeName=Value|Tim_gen|CAN_ID  AttributeFrom=Signal port|Signal port|Dialog  AttributeValue=1|1|CAN_ID  AttributeTreatAsVector=1|1|1  EvaluatedAttributeValue={ [];[];CAN_ID}
      settings: InputPortMap=u0,u1
  Time-Based Entity Generator : TimeBasedEntityGenerator  Distribution=Uniform  Period=Tint  Minimum=Tint  Maximum=Tint+0.1
  Timed to Event Signal : TimedToEventSignal
  Timed to Event Signal1 : TimedToEventSignal
  TX : PMIOPort  Port=1  Side=Right
  RX : PMIOPort  Port=2  Side=Left
  Out1 : Outport
  wires:
  Quantizer/1 -> Timed to Event Signal/1
  Timed to Event Signal/1 -> Set Attribute/1
  Clock/1 -> Timed to Event Signal1/1
  Timed to Event Signal1/1 -> Set Attribute/2
  Constant1/1 -> Quantizer/1
  Get Attribute/2 -> Event to Timed Signal1/1
  Get Attribute/1 -> Event to Timed Signal/1
  Get Attribute1/1 -> Event to Timed Signal2/1
  Get Attribute1/2 -> Event to Timed Signal3/1
  Get Attribute2/1 -> Event to Timed Signal4/1
  Get Attribute2/2 -> Event to Timed Signal5/1
  Event to Timed Signal/1 -> Multiport Switch/2
  Event to Timed Signal2/1 -> Multiport Switch/3
  Event to Timed Signal4/1 -> Multiport Switch/4
  Accepted ID/1 -> Multiport Switch/1
  Multiport Switch/1 -> Memory/1
  Memory/1 -> Out1/1
  connections:
  Set Attribute/RConn1 -- FIFO Queue/LConn1
  FIFO Queue/RConn1 -- TX/RConn1
  RX/RConn1 -- Output Switch/LConn1
  Output Switch/RConn1 -- Get Attribute/LConn1
  Get Attribute1/LConn1 -- Output Switch/RConn2
  Get Attribute2/LConn1 -- Output Switch/RConn3
  Get Attribute2/RConn1 -- Entity Sink/LConn1
  Get Attribute/RConn1 -- Entity Sink2/LConn1
  Get Attribute1/RConn1 -- Entity Sink1/LConn1
  Time-Based Entity Generator/RConn1 -- Set Attribute/LConn1

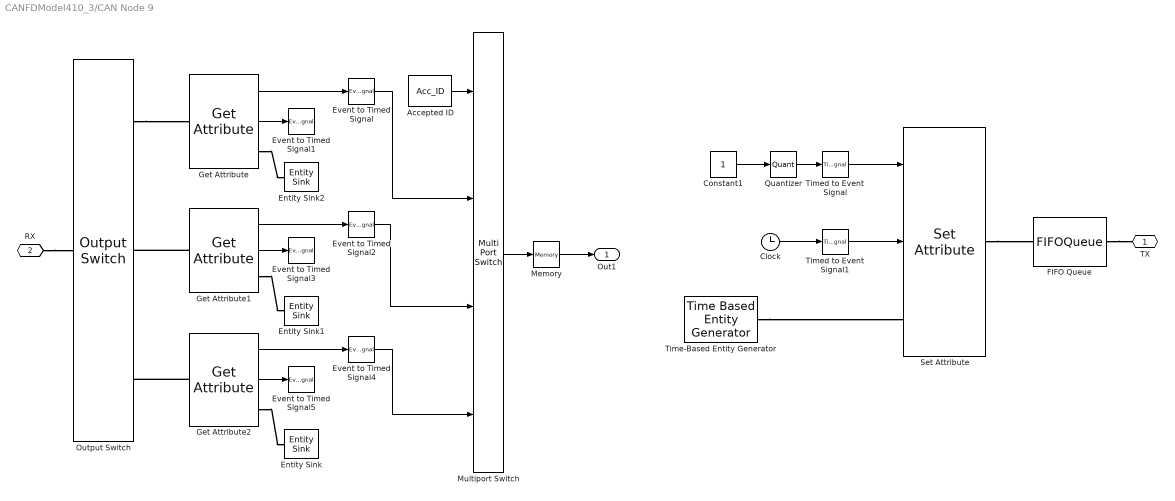
== system CANFDModel410_3/CAN Node 9 ==
  Accepted ID : Constant  Value=Acc_ID
  Clock : Clock
  Constant1 : Constant
  Entity Sink : EntitySink
  Entity Sink1 : EntitySink
  Entity Sink2 : EntitySink
  Event to Timed Signal{,1..5} (6 alike) : EventToTimedSignal
  FIFO Queue : FIFOQueue  Capacity=3
  Get Attribute : GetAttribute  AttributeName=Value|CAN_ID  AttributeMissing=Error|Error  AttributeDefaultValue=1|1  AttributeTreatAsVector=1|1  AttributeSendTiming=After entity departure|After entity departure  EvaluatedDefaultAttributeValue={ [];[]}
      settings: OutputPortMap=o1,o2
  Get Attribute1 : GetAttribute  AttributeName=Value|CAN_ID  AttributeMissing=Error|Error  AttributeDefaultValue=1|1  AttributeTreatAsVector=1|1  AttributeSendTiming=After entity departure|After entity departure  EvaluatedDefaultAttributeValue={ [];[]}
      settings: OutputPortMap=o1,o2
  Get Attribute2 : GetAttribute  AttributeName=Value|CAN_ID  AttributeMissing=Error|Error  AttributeDefaultValue=1|1  AttributeTreatAsVector=1|1  AttributeSendTiming=After entity departure|After entity departure  EvaluatedDefaultAttributeValue={ [];[]}
      settings: OutputPortMap=o1,o2
  Memory : Memory
  Multiport Switch : MultiPortSwitch
  Output Switch : OutputSwitch
  Quantizer : Quantizer  QuantizationInterval=(MAXM-MINM)/2^bitlength%%800/2^16%%
  Set Attribute : SetAttribute  AttributeName=Value|Tim_gen|CAN_ID  AttributeFrom=Signal port|Signal port|Dialog  AttributeValue=1|1|CAN_ID  AttributeTreatAsVector=1|1|1  EvaluatedAttributeValue={ [];[];CAN_ID}
      settings: InputPortMap=u0,u1
  Time-Based Entity Generator : TimeBasedEntityGenerator  Distribution=Uniform  Period=Tint  Minimum=Tint  Maximum=Tint+0.1
  Timed to Event Signal : TimedToEventSignal
  Timed to Event Signal1 : TimedToEventSignal
  TX : PMIOPort  Port=1  Side=Right
  RX : PMIOPort  Port=2  Side=Left
  Out1 : Outport
  wires:
  Memory/1 -> Out1/1
  Multiport Switch/1 -> Memory/1
  Accepted ID/1 -> Multiport Switch/1
  Event to Timed Signal4/1 -> Multiport Switch/4
  Event to Timed Signal2/1 -> Multiport Switch/3
  Event to Timed Signal/1 -> Multiport Switch/2
  Get Attribute2/2 -> Event to Timed Signal5/1
  Get Attribute2/1 -> Event to Timed Signal4/1
  Get Attribute1/2 -> Event to Timed Signal3/1
  Get Attribute1/1 -> Event to Timed Signal2/1
  Get Attribute/1 -> Event to Timed Signal/1
  Get Attribute/2 -> Event to Timed Signal1/1
  Constant1/1 -> Quantizer/1
  Timed to Event Signal1/1 -> Set Attribute/2
  Clock/1 -> Timed to Event Signal1/1
  Timed to Event Signal/1 -> Set Attribute/1
  Quantizer/1 -> Timed to Event Signal/1
  connections:
  Get Attribute1/RConn1 -- Entity Sink1/LConn1
  Get Attribute/RConn1 -- Entity Sink2/LConn1
  Get Attribute2/RConn1 -- Entity Sink/LConn1
  Get Attribute2/LConn1 -- Output Switch/RConn3
  Get Attribute1/LConn1 -- Output Switch/RConn2
  Output Switch/RConn1 -- Get Attribute/LConn1
  RX/RConn1 -- Output Switch/LConn1
  FIFO Queue/RConn1 -- TX/RConn1
  Time-Based Entity Generator/RConn1 -- Set Attribute/LConn1
  Set Attribute/RConn1 -- FIFO Queue/LConn1
